simulink model "SerialFrame"  (R2025b)
settings: Solver=FixedStepAuto  StartTime=0.0  StopTime=10  FixedStep=0.0002  RelTol=1e-3
undefined symbols (not defined in the file or in its folder): CR, LF
libraries: instrumentseriallib x2, svdutilitieslib x2
settings Model: VariantFading=off  Creator=Akkarasaknarong  LastModifiedBy=Akkarasaknarong

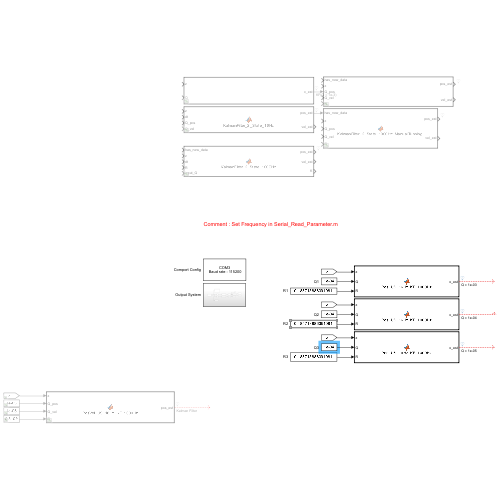
[thumbnail: Simulink's stored preview of the top-level diagram]
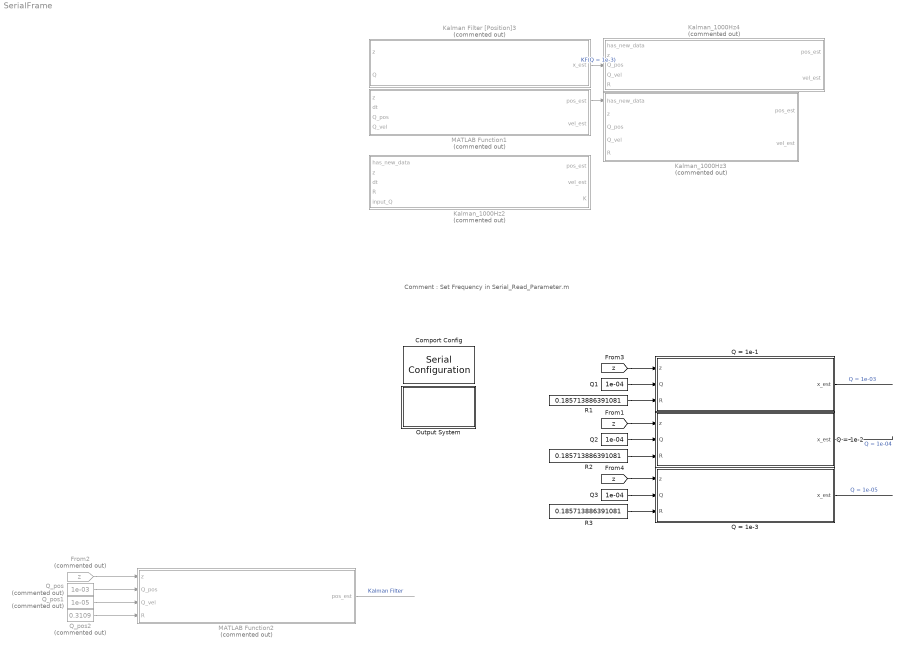
== system SerialFrame ==
  note: Comment : Set Frequency in Serial_Read_Parameter.m
  Comport Config : instrumentseriallib/Serial Configuration  Priority=-200000  PortSel=COM3  Port=COM3  ComPort=COM3  BaudRate=115200  DataBits=8  Parity=none  StopBits=1  ByteOrder=little-endian  FlowControl=none  Timeout=10  SimulateUsing=Interpreted execution  BlockInModel=on  aMode=1
      settings: LibrarySourceBlock=embeddedtargetslib/Host Communication/Serial Configuration
  From2 : From  Commented=on  GotoTag=z  TagVisibility=global
  Kalman Filter [Position]3 : MATLAB Function  Commented=on  TreatAsAtomicUnit=on
  Kalman_1000Hz2 : MATLAB Function  Commented=on  TreatAsAtomicUnit=on
  Kalman_1000Hz3 : MATLAB Function  Commented=on  TreatAsAtomicUnit=on
  Kalman_1000Hz4 : MATLAB Function  Commented=on  TreatAsAtomicUnit=on
  MATLAB Function1 : MATLAB Function  Commented=on  TreatAsAtomicUnit=on
  MATLAB Function2 : MATLAB Function  Commented=on  TreatAsAtomicUnit=on
  Output System : Subsystem
  Q = 1e-1 : MATLAB Function  TreatAsAtomicUnit=on
  Q = 1e-2 : MATLAB Function  TreatAsAtomicUnit=on
  Q = 1e-3 : MATLAB Function  TreatAsAtomicUnit=on
  Q1 : Constant  Value=1e-04
  Q2 : Constant  Value=1e-04
  Q3 : Constant  Value=1e-04
  Q_pos : Constant  Commented=on  Value=1e-03
  Q_pos1 : Constant  Commented=on  Value=1e-05
  Q_pos2 : Constant  Commented=on  Value=0.3109
  R1 : Constant  Value=0.185713886391081
  R2 : Constant  Value=0.185713886391081
  R3 : Constant  Value=0.185713886391081
  wires:
  [z] -> Q = 1e-1/1(z)
  Q = 1e-1/1(x_est) -> ?  "Q = 1e-03"
  R1/1 -> Q = 1e-1/3(R)
  Q1/1 -> Q = 1e-1/2(Q)
  MATLAB Function1/1(pos_est) -> Kalman_1000Hz3/1(has_new_data)
  Kalman Filter [Position]3/1(x_est) -> Kalman_1000Hz4/3(Q_pos)  "KF(Q = 1e-3)"
  MATLAB Function2/1(pos_est) -> ?  "Kalman Filter"
  Q_pos/1 -> MATLAB Function2/2(Q_pos)
  Q_pos1/1 -> MATLAB Function2/3(Q_vel)
  Q_pos2/1 -> MATLAB Function2/4(R)
  From2/1 -> MATLAB Function2/1(z)
  R2/1 -> Q = 1e-2/3(R)
  Q = 1e-2/1(x_est) -> ?  "Q = 1e-04"
  Q2/1 -> Q = 1e-2/2(Q)
  [z] -> Q = 1e-2/1(z)
  Q3/1 -> Q = 1e-3/2(Q)
  [z] -> Q = 1e-3/1(z)
  Q = 1e-3/1(x_est) -> ?  "Q = 1e-05"
  R3/1 -> Q = 1e-3/3(R)

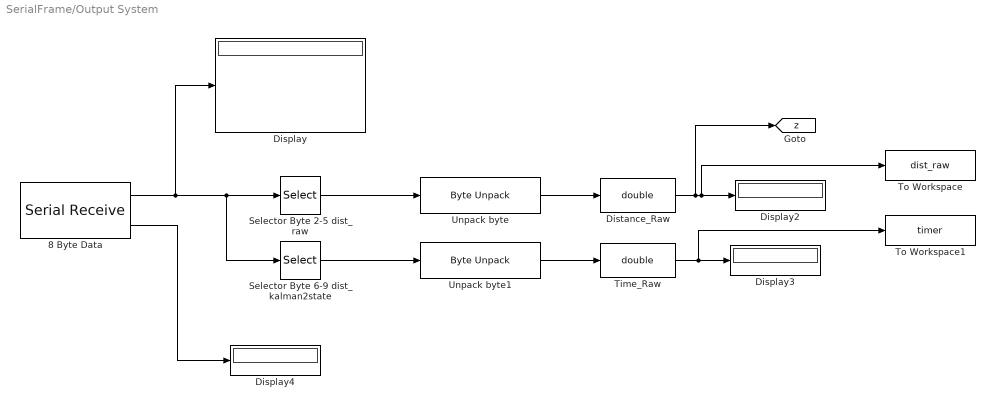
== system SerialFrame/Output System ==
  8 Byte Data : instrumentseriallib/Serial Receive  Priority=1  PortSel=COM3  Port=COM3  ComPort=COM3  DataType=uint8  SaveDataType=uint8  ToggleHeader=on  Header=[170 85]  ToggleDataSize=on  DataSize=[10 1]  ToggleTerminator=off  Terminator=CR/LF ('\r\n')  CustomTerminator=[]  InputFormat=Column major  EnableBlockingMode=off  ActionDataUnavailable=Output last received value  ActionWhenDataUnavailable=Output last received value  CustomValue=-50  SampleTime=0.001  SimulateUsing=Interpreted execution  BlockInModel=on  aMode=1  LibraryInUse=instrumentlib
      settings: LibrarySourceBlock=embeddedtargetslib/Host Communication/Serial Receive
  Display{,2..4} (4 alike) : Display
  Distance_Raw : DataTypeConversion  OutDataTypeStr=double  SaturateOnIntegerOverflow=off  RndMeth=Floor
  Selector Byte 2-5 dist_raw : Selector  InputPortWidth=10  IndexOptions=Index vector (dialog)  Indices=[2 3 4 5]  OutputSizes=1
  Selector Byte 6-9 dist_kalman2state : Selector  InputPortWidth=10  IndexOptions=Index vector (dialog)  Indices=[6 7 8 9]  OutputSizes=1
  Time_Raw : DataTypeConversion  OutDataTypeStr=double  SaturateOnIntegerOverflow=off  RndMeth=Floor
  To Workspace : ToWorkspace  VariableName=dist_raw  SaveFormat=Timeseries  SampleTime=-1
  To Workspace1 : ToWorkspace  VariableName=timer  SaveFormat=Timeseries  SampleTime=-1
  Unpack byte : svdutilitieslib/Byte Unpack  dimensions={[1]}  datatypes={'single'}  byteAlign=1  blockPlatform=arduinoert
      settings: LibrarySourceBlock=mcblib/Signal Management/Byte Unpack
  Unpack byte1 : svdutilitieslib/Byte Unpack  dimensions={[1]}  datatypes={'single'}  byteAlign=1  blockPlatform=arduinoert
      settings: LibrarySourceBlock=mcblib/Signal Management/Byte Unpack
  tag scope: z=global
  wires:
  Unpack byte/1 -> Distance_Raw/1
  8 Byte Data/1 -> Display/1, Selector Byte 6-9 dist_kalman2state/1, Selector Byte 2-5 dist_raw/1
  Selector Byte 2-5 dist_raw/1 -> Unpack byte/1
  Selector Byte 6-9 dist_kalman2state/1 -> Unpack byte1/1
  Unpack byte1/1 -> Time_Raw/1
  Distance_Raw/1 -> [z], To Workspace/1, Display2/1
  Time_Raw/1 -> To Workspace1/1, Display3/1
  8 Byte Data/2 -> Display4/1

== matlab function SerialFrame/MATLAB Function1 ==
  data: z input; pos_est output; dt input; Q_pos input; Q_vel input; vel_est output
function [pos_est,vel_est] = KalmanFilter_2_State_16Hz(z,dt,Q_pos,Q_vel)

% Define Variable
persistent x_prev p_prev ;
R = 2.92e-3;

if isempty(x_prev)
    x_prev = [0;0];
end
if isempty(p_prev)
    p_prev = eye(2);
end


% Define Matrix
F = [1 dt;
     0 1 ];
H = [1 0];
Q = [Q_pos 0;
     0     Q_vel];

% State 1: Prediction State
x_pred = F * x_prev ;
p_pred = (F*p_prev*F') + Q ;

% State 2: Correction State
K = (p_pred * H') / (H * p_pred * H' + R) ; 
error = z - H * x_pred ;
x_est = x_pred + (K * error);
p_est = (eye(2) - K*H)*p_pred ;

p_prev = p_est ;
x_prev = x_est ;

pos_est = x_est(1);
vel_est = x_est(2);

== matlab function SerialFrame/Kalman_1000Hz4 ==
  data: has_new_data input; z input; pos_est output; Q_pos input; Q_vel input; vel_est output; R input
function [pos_est,vel_est] = KalmanFilter_2_State_1000Hz_ManualTunning(has_new_data,z,Q_pos,Q_vel,R)
k = 29.839 ;
b = 0.0102;
m = 0.195 ;
g = 9.81 ;
dt = 0.001 ;

% Define Variable
persistent x_prev p_prev z_prev;
if isempty(x_prev)
    x_prev = [0;0];
end
if isempty(p_prev)
    p_prev = eye(2);
end
if isempty(z_prev)
    z_prev = 0 ;
end

% Define Matrix
% F = [0 1;
%      k/m b/m];

F = [ 1            ,  dt; 
     -(k/m)*dt     ,  1 - (b/m)*dt ];

H = [1 0];

Q = [Q_pos 0;
     0     Q_vel];

z_equilibrium = 9.06;
z = z- z_equilibrium ;

% State 1: Prediction State
x_pred = F * x_prev ;
p_pred = (F*p_prev*F') + Q ;

% State 2: Correction State
if has_new_data 
    K = (p_pred * H') / (H * p_pred * H' + R) ; 
    error = z - H * x_pred ;
    x_est = x_pred + (K * error);
    p_est = (eye(2) - K*H)*p_pred ;
else
    x_est = x_pred ;
    p_est = p_pred ;
end

p_prev = p_est ;
x_prev = x_est ;
z_prev = z ;

pos_est = x_est(1) + z_equilibrium;
vel_est = x_est(2);

== matlab function SerialFrame/Q = 1e-2 ==
  data: z input; x_est output; Q input; R input
function x_est = Pos_US_16Hz_KF_1000Hz(z,Q,R)
% State 1: Prediction state
persistent x_prev  p_prev;
if isempty(x_prev)
    x_prev = 0 ;
end
if isempty(p_prev)
    p_prev = R ; % 50% trust in model and sensor
end

x_pred = x_prev ;       % Predict x
p_pred = p_prev + Q ;   % Predict p

% State 2: Correction state
K = p_pred /(p_pred + R);  % Compute Kalman Gain (Trust model or sensor)
error = z - x_pred ;
x_est = x_pred + (K*error); % Estimate x
p_est = (1 - K)*p_pred ; % check should confident in model

x_prev = x_est;
p_prev = p_est;

== matlab function SerialFrame/Kalman Filter [Position]3 ==
  data: z input; x_est output; Q input
function x_est = KalmanFilter_1_State_16Hz(z,Q)
R = 2.92e-3 ;

% State 1: Prediction state
persistent x_prev  p_prev;
if isempty(x_prev)
    x_prev = 0 ;
end
if isempty(p_prev)
    p_prev = (0.5*R)/0.5 ; % 50% trust in model and sensor
end

x_pred = x_prev ;       % Predict x
p_pred = p_prev + Q ;   % Predict p


% State 2: Correction state
K = p_pred /(p_pred + R);  % Compute Kalman Gain (Trust model or sensor)

error = z - x_pred ;
x_est = x_pred + (K*error); % Estimate x 

p_est = (1 - K)*p_pred ; % check should confident in model

x_prev = x_est;
p_prev = p_est;

== matlab function SerialFrame/Q = 1e-3 ==
  data: z input; x_est output; Q input; R input
function x_est = Pos_US_16Hz_KF_1000Hz(z,Q,R)
% State 1: Prediction state
persistent x_prev  p_prev;
if isempty(x_prev)
    x_prev = 0 ;
end
if isempty(p_prev)
    p_prev = R ; % 50% trust in model and sensor
end

x_pred = x_prev ;       % Predict x
p_pred = p_prev + Q ;   % Predict p

% State 2: Correction state
K = p_pred /(p_pred + R);  % Compute Kalman Gain (Trust model or sensor)
error = z - x_pred ;
x_est = x_pred + (K*error); % Estimate x
p_est = (1 - K)*p_pred ; % check should confident in model

x_prev = x_est;
p_prev = p_est;

== matlab function SerialFrame/Kalman_1000Hz2 ==
  data: has_new_data input; z input; pos_est output; dt input; vel_est output; K output; R input; input_Q input
function [pos_est,vel_est,K] = KalmanFilter_2_State_1000Hz(has_new_data,z,dt,R,input_Q)

% Define Variable
persistent x_prev p_prev z_prev K_prev;
if isempty(x_prev)
    x_prev = [0;0];
end
if isempty(p_prev)
    p_prev = eye(2);
end
if isempty(z_prev)
    z_prev = 0 ;
end
if isempty(K_prev)
    K_prev = [0;0];
end


% Define Matrix
F = [1 dt;
     0 1 ];
H = [1 0];

Q = input_Q * [ (dt^4)/4 , (dt^3)/2 ; 
                   (dt^3)/2 ,   dt^2   ];

% State 1: Prediction State
x_pred = F * x_prev ;
p_pred = (F*p_prev*F') + Q ;

% State 2: Correction State
if has_new_data 
    K = (p_pred * H') / (H * p_pred * H' + R) ; 
    error = z - H * x_pred ;
    x_est = x_pred + (K * error);
    p_est = (eye(2) - K*H)*p_pred ;
    K_prev = K;
else
    x_est = x_pred ;
    p_est = p_pred ;
    K = K_prev;
end

p_prev = p_est ;
x_prev = x_est ;
z_prev = z ;

pos_est = x_est(1);
vel_est = x_est(2);

== matlab function SerialFrame/Kalman_1000Hz3 ==
  data: has_new_data input; z input; pos_est output; Q_pos input; Q_vel input; vel_est output; R input
function [pos_est,vel_est] = KalmanFilter_2_State_1000Hz_ManualTunning(has_new_data,z,Q_pos,Q_vel,R)
k = 29.839 ;
b = 0.0102;
m = 0.195 ;
g = 9.81 ;
dt = 0.001 ;

% Define Variable
persistent x_prev p_prev z_prev;
if isempty(x_prev)
    x_prev = [0;0];
end
if isempty(p_prev)
    p_prev = eye(2);
end
if isempty(z_prev)
    z_prev = 0 ;
end

% Define Matrix
% F = [0 1;
%      k/m b/m];

F = [ 1            ,  dt; 
     -(k/m)*dt     ,  1 - (b/m)*dt ];

H = [1 0];

Q = [Q_pos 0;
     0     Q_vel];

z_equilibrium = 9.06;
z = z- z_equilibrium ;

% State 1: Prediction State
x_pred = F * x_prev ;
p_pred = (F*p_prev*F') + Q ;

% State 2: Correction State
if has_new_data 
    K = (p_pred * H') / (H * p_pred * H' + R) ; 
    error = z - H * x_pred ;
    x_est = x_pred + (K * error);
    p_est = (eye(2) - K*H)*p_pred ;
else
    x_est = x_pred ;
    p_est = p_pred ;
end

p_prev = p_est ;
x_prev = x_est ;
z_prev = z ;

pos_est = x_est(1) + z_equilibrium;
vel_est = x_est(2);

== matlab function SerialFrame/MATLAB Function2 ==
  data: z input; Q_pos input; pos_est output; Q_vel input; R input
function pos_est  = PosVel_US_16Hz_KF_1000Hz(z,Q_pos,Q_vel,R)
dt = 0.001 ;

% Define Variable
persistent x_prev p_prev ;
if isempty(x_prev)
    x_prev = [0;0];
end
if isempty(p_prev)
    p_prev = eye(2);
end

% Define Matrix
F = [1 dt;
     0 1 ];
H = [1 0];
Q = [Q_pos 0;
     0     Q_vel];

% State 1: Prediction State
x_pred = F * x_prev ;
p_pred = (F*p_prev*F') + Q ;

% State 2: Correction State

K = (p_pred * H') / (H * p_pred * H' + R) ; 
error = z - H * x_pred ;
x_est = x_pred + (K * error);
p_est = (eye(2) - K*H)*p_pred ;

p_prev = p_est ;
x_prev = x_est ;
pos_est = x_est(1);

== matlab function SerialFrame/Q = 1e-1 ==
  data: z input; x_est output; Q input; R input
function x_est = Pos_US_16Hz_KF_1000Hz(z,Q,R)
% State 1: Prediction state
persistent x_prev  p_prev;
if isempty(x_prev)
    x_prev = 0 ;
end
if isempty(p_prev)
    p_prev = R ; % 50% trust in model and sensor
end

x_pred = x_prev ;       % Predict x
p_pred = p_prev + Q ;   % Predict p

% State 2: Correction state
K = p_pred /(p_pred + R);  % Compute Kalman Gain (Trust model or sensor)
error = z - x_pred ;
x_est = x_pred + (K*error); % Estimate x
p_est = (1 - K)*p_pred ; % check should confident in model

x_prev = x_est;
p_prev = p_est;
